simulink model "SpeedController"  (Simulink 7.6)
settings: Solver=ode45  StartTime=0.0  StopTime=10.0  RelTol=1e-3
libraries: simulink x1
settings Model: Creator=Zsolt  LastModifiedBy=bapty
settings HardwareCC: TargetIntDivRoundTo=Zero  TargetEndianess=LittleEndian  TargetHWDeviceType=MATLAB Host  ProdEqTarget=off
settings RTWCC: SystemTargetFile=rsim.tlc  TemplateMakefile=rsim_default_tmf  Description=Rapid Simulation Target  ProcessScript=rsim_make_rtw_hook
settings RSimTargetCC: TargetFunctionLibrary=ANSI_C  ERTMultiwordTypeDef=System defined  ERTCodeCoverageTool=None  ERTMultiwordLength=256  IsPILTarget=off  EnableShiftOperators=on  PortableWordSizes=off

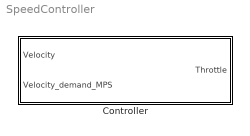
== system SpeedController ==
  Controller : Subsystem

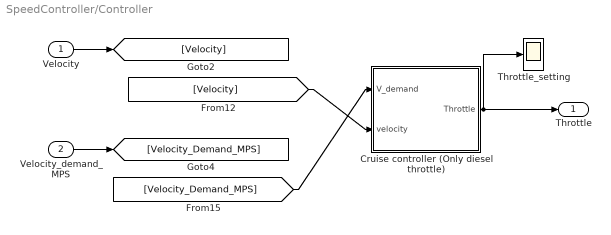
== system SpeedController/Controller ==
  Velocity : Inport
  Velocity_demand_MPS : Inport  Port=2
  Cruise controller (Only diesel throttle) : Subsystem
  Throttle_setting : Scope
      settings: TimeRange=500  YMin=0  YMax=1  SaveName=ScopeData4
  Throttle : Outport
  wires:
  Cruise controller (Only diesel throttle)/1(Throttle) -> Throttle_setting/1, Throttle/1
  [Velocity] -> Cruise controller (Only diesel throttle)/2(velocity)
  [Velocity_Demand_MPS] -> Cruise controller (Only diesel throttle)/1(V_demand)
  Velocity/1 -> [Velocity]
  Velocity_demand_MPS/1 -> [Velocity_Demand_MPS]

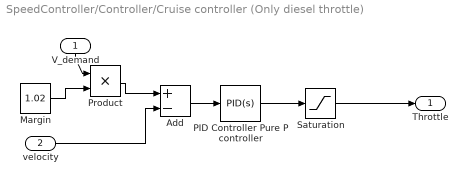
== system SpeedController/Controller/Cruise controller (Only diesel throttle) ==
  V_demand : Inport
  velocity : Inport  Port=2
  Add : Sum  Inputs=+-
  Margin : Constant  Value=1.02
  PID Controller Pure P controller : simulink/Continuous/PID Controller  DialogController=pidpack.PIDConfig.pidDDGCreate  DialogControllerArgs=DataTag0  SystemSampleTime=-1  Controller=PID  TimeDomain=Continuous-time  SampleTime=1  IntegratorMethod=Forward Euler  FilterMethod=Forward Euler  Form=Parallel  P=7  I=0  D=0  N=100  InitialConditionSource=internal  InitialConditionForIntegrator=0  InitialConditionForFilter=0  ExternalReset=none  LimitOutput=off  UpperSaturationLimit=inf  LowerSaturationLimit=-inf  LinearizeAsGain=off  AntiWindupMode=none  Kb=1  TrackingMode=off  Kt=1  PParamMin=[]  PParamMax=[]  IParamMin=[]  IParamMax=[]  DParamMin=[]  DParamMax=[]  NParamMin=[]  NParamMax=[]  KbParamMin=[]  KbParamMax=[]  KtParamMin=[]  KtParamMax=[]  POutMin=[]  POutMax=[]  IOutMin=[]  IOutMax=[]  DOutMin=[]  DOutMax=[]  NOutMin=[]  NOutMax=[]  KbOutMin=[]  KbOutMax=[]  KtOutMin=[]  KtOutMax=[]  IntegratorOutMin=[]  IntegratorOutMax=[]  FilterOutMin=[]  FilterOutMax=[]  SumOutMin=[]  SumOutMax=[]  SumI1OutMin=[]  SumI1OutMax=[]  SumI2OutMin=[]  SumI2OutMax=[]  SumI3OutMin=[]  SumI3OutMax=[]  SumDOutMin=[]  SumDOutMax=[]  SaturationOutMin=[]  SaturationOutMax=[]  IntegratorContinuousStateAttributes=''  IntegratorStateMustResolveToSignalObject=off  IntegratorRTWStateStorageClass=Auto  FilterContinuousStateAttributes=''  FilterStateMustResolveToSignalObject=off  FilterRTWStateStorageClass=Auto
  Product : Product  RndMeth=Zero
  Saturation : Saturate  UpperLimit=1  LowerLimit=0
  Throttle : Outport
  wires:
  Product/1 -> Add/1
  Add/1 -> PID Controller Pure P controller/1
  PID Controller Pure P controller/1 -> Saturation/1
  V_demand/1 -> Product/1
  velocity/1 -> Add/2
  Saturation/1 -> Throttle/1
  Margin/1 -> Product/2
